simulink model "Damper_Bicycle_Output_Dec1"  (R2020a)
settings: Solver=ode4  StartTime=0.0  StopTime=2  FixedStep=0.0005  RelTol=1e-3  EnableMultiTasking=on
settings Model: Creator=Cason  LastModifiedBy=mjmck
settings SolverCC: AlgebraicLoopSolver=LineSearch

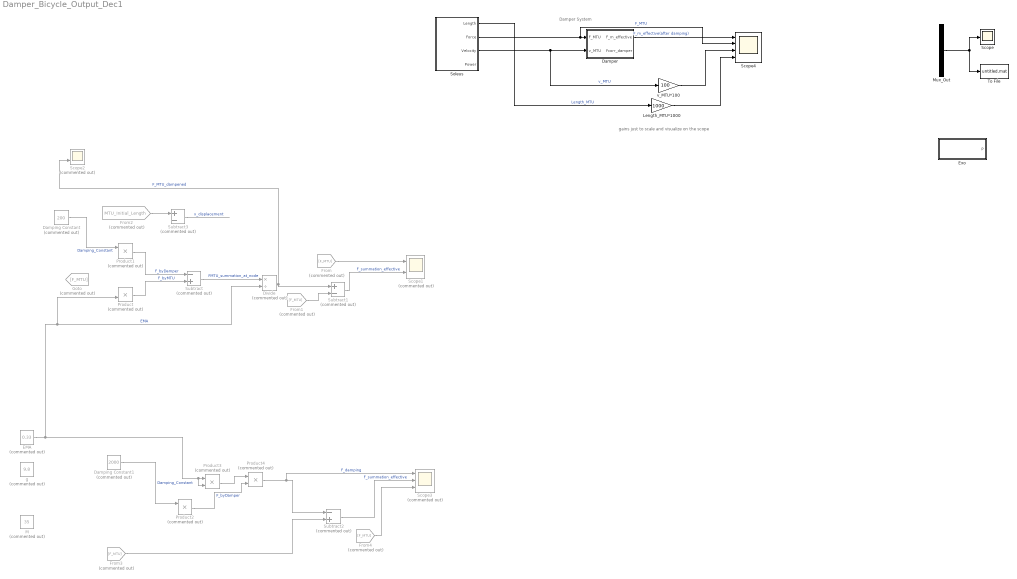
== system Damper_Bicycle_Output_Dec1 ==
  note: gains just to scale and visualize on the scope
  note: Damper System
  Damper : Subsystem
  Damping Constant : Constant  Commented=on  Value=200
  Damping Constant1 : Constant  Commented=on  Value=2000
  Divide : Product  Commented=on  Inputs=*/
  EMA : Constant  Commented=on  Value=0.33
  Exo : Subsystem
  From{,1,3..4} (4 alike) : From  Commented=on  GotoTag=F_MTU
  From2 : From  Commented=on  GotoTag=MTU_Initial_Length  TagVisibility=global
  Goto : Goto  Commented=on  GotoTag=F_MTU
  Length_MTU*1000 : Gain  Gain=1000
  M : Constant  Commented=on  Value=35
  Mux_Out : Mux
  Product{,1..4} (5 alike) : Product  Commented=on
  Scope : Scope
  Scope1 : Scope  Commented=on  NumInputPorts=2
  Scope2 : Scope  Commented=on  NumInputPorts=2
  Scope3 : Scope  Commented=on  NumInputPorts=3
  Scope4 : Scope  NumInputPorts=4
  Soleus : Subsystem
  Subtract : Sum  Commented=on  Inputs=-+
  Subtract1 : Sum  Commented=on  Inputs=+-
  Subtract2 : Sum  Commented=on  Inputs=-+
  Subtract3 : Sum  Commented=on  Inputs=+-
  To File : ToFile  MatrixName=out
  g : Constant  Commented=on  Value=9.8
  v_MTU*100 : Gain  Gain=100
  wires:
  Mux_Out/1 -> To File/1, Scope/1
  ? -> Scope2/1, Product/1, Goto/1  "F_MTU"
  EMA/1 -> Product3/2, Product3/1, Divide/2, Product/2  "EMA"
  Product/1 -> Subtract/2  "F_byMTU"
  ? -> Product2/2, Product1/2  "v_MTU"
  Product1/1 -> Subtract/1  "F_byDamper"
  Damping Constant/1 -> Product1/1  "Damping_Constant"
  Subtract/1 -> Divide/1  "FMTU_summation_at_node"
  Divide/1 -> Subtract1/1, Scope2/2  "F_MTU_dampened"
  From/1 -> Scope1/1
  From1/1 -> Subtract1/2
  Subtract1/1 -> Scope1/2  "F_summation_effective"
  ? -> Subtract3/2
  From2/1 -> Subtract3/1
  Subtract3/1 -> ?  "x_displacement"
  From3/1 -> Subtract2/2
  Damping Constant1/1 -> Product2/1  "Damping_Constant"
  Subtract2/1 -> Scope3/2  "F_summation_effective"
  From4/1 -> Scope3/3
  Product3/1 -> Product4/1
  Product2/1 -> Product4/2  "F_byDamper"
  Product4/1 -> Scope3/1, Subtract2/1  "F_damping"
  Soleus/3(Velocity) -> v_MTU*100/1, Damper/2(v_MTU)  "v_MTU"
  Soleus/2(Force) -> Scope4/2, Damper/1(F_MTU)  "F_MTU"
  Damper/1(F_m_effective) -> Scope4/1  "F_m_effective(after damping)"
  Soleus/1(Length) -> Length_MTU*1000/1  "Length_MTU"
  Length_MTU*1000/1 -> Scope4/4
  v_MTU*100/1 -> Scope4/3

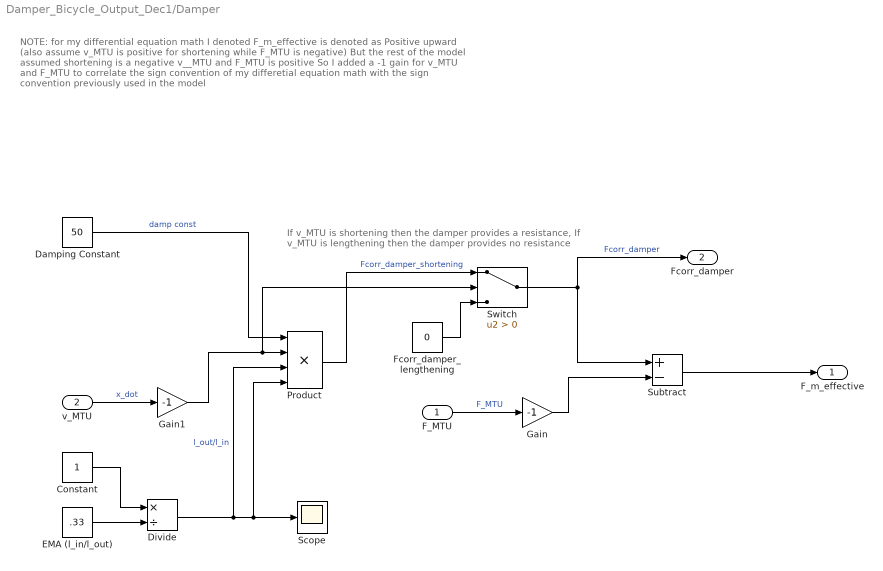
== system Damper_Bicycle_Output_Dec1/Damper ==
  note: NOTE:
      | for my differential equation math I denoted
      | 	F_m_effective is denoted as Positive upward (also assume v_MTU is positive for 			shortening while F_MTU is negative)
      |
      | But the rest of the model assumed shortening is a negative v__MTU and F_MTU is positive
      |
      | So I added a -1 gain for v_MTU and F_MTU to correlate the sign convention of my differetial equation math with the sign convention previously used in the model
  note: If v_MTU is shortening then the damper provides a resistance,
      | If v_MTU is lengthening then the damper provides no resistance
  F_MTU : Inport
  v_MTU : Inport  Port=2
  Constant : Constant
  Damping Constant : Constant  Value=50
  Divide : Product  Inputs=*/
  EMA (l_in/l_out) : Constant  Value=.33
  Fcorr_damper_lengthening : Constant  Value=0
  Gain : Gain  Gain=-1
  Gain1 : Gain  Gain=-1
  Product : Product  Inputs=4
  Scope : Scope
  Subtract : Sum  Inputs=+-
  Switch : Switch  Criteria=u2 > Threshold
  F_m_effective : Outport
  Fcorr_damper : Outport  Port=2
  wires:
  F_MTU/1 -> Gain/1  "F_MTU"
  Damping Constant/1 -> Product/1  "damp const"
  v_MTU/1 -> Gain1/1  "x_dot"
  EMA (l_in/l_out)/1 -> Divide/2
  Product/1 -> Switch/1  "Fcorr_damper_shortening"
  Constant/1 -> Divide/1
  Divide/1 -> Product/3, Product/4, Scope/1  "l_out/l_in"
  Switch/1 -> Fcorr_damper/1, Subtract/1  "Fcorr_damper"
  Fcorr_damper_lengthening/1 -> Switch/3
  Subtract/1 -> F_m_effective/1
  Gain/1 -> Subtract/2
  Gain1/1 -> Switch/2, Product/2

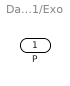
== system Damper_Bicycle_Output_Dec1/Exo ==
  P : Outport

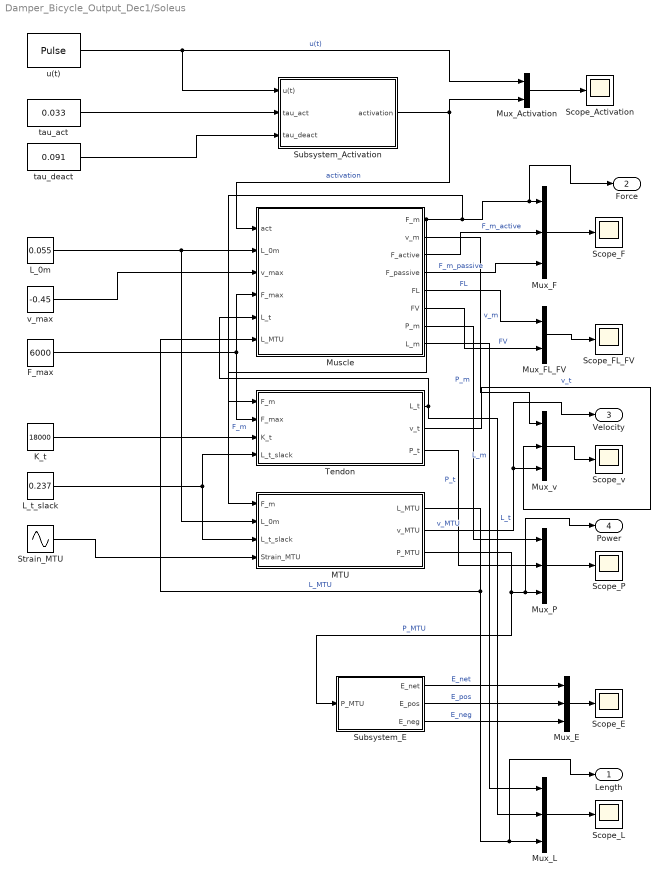
== system Damper_Bicycle_Output_Dec1/Soleus ==
  F_max : Constant  Value=6000
  K_t : Constant  Value=18000
  L_0m : Constant  Value=0.055
  L_t_slack : Constant  Value=0.237
  MTU : Subsystem
  Muscle : Subsystem
  Mux_Activation : Mux  Inputs=2
  Mux_E : Mux  Inputs=3
  Mux_F : Mux  Inputs=3
  Mux_FL_FV : Mux  Inputs=2
  Mux_L : Mux  Inputs=3
  Mux_P : Mux  Inputs=3
  Mux_v : Mux  Inputs=3
  Scope_Activation : Scope
  Scope_E : Scope
  Scope_F : Scope
  Scope_FL_FV : Scope
  Scope_L : Scope
  Scope_P : Scope
  Scope_v : Scope
  Strain_MTU : Sin  Amplitude=0.05  Bias=1  Frequency=5*pi  SampleTime=0
  Subsystem_Activation : Subsystem
  Subsystem_E : Subsystem
  Tendon : Subsystem
  tau_act : Constant  Value=0.033
  tau_deact : Constant  Value=0.091
  u(t) : DiscretePulseGenerator  PulseType=Time based  Period=0.4  PulseWidth=10
  v_max : Constant  Value=-0.45
  Length : Outport
  Force : Outport  Port=2
  Velocity : Outport  Port=3
  Power : Outport  Port=4
  wires:
  Mux_v/1 -> Scope_v/1
  u(t)/1 -> Mux_Activation/1, Subsystem_Activation/1(u(t))  "u(t)"
  Muscle/7(P_m) -> Mux_P/1  "P_m"
  tau_act/1 -> Subsystem_Activation/2(tau_act)
  K_t/1 -> Tendon/3(K_t)
  Mux_F/1 -> Scope_F/1
  MTU/3(P_MTU) -> Subsystem_E/1(P_MTU), Power/1, Mux_P/3  "P_MTU"
  Tendon/2(v_t) -> Mux_v/2  "v_t"
  L_t_slack/1 -> MTU/3(L_t_slack), Tendon/4(L_t_slack)
  MTU/1(L_MTU) -> Length/1, Mux_L/3, Muscle/6(L_MTU)  "L_MTU"
  Mux_P/1 -> Scope_P/1
  Tendon/1(L_t) -> Mux_L/2, Muscle/5(L_t)  "L_t"
  Mux_Activation/1 -> Scope_Activation/1
  MTU/2(v_MTU) -> Velocity/1, Mux_v/3  "v_MTU"
  Strain_MTU/1 -> MTU/4(Strain_MTU)
  Muscle/8(L_m) -> Mux_L/1  "L_m"
  Muscle/5(FL) -> Mux_FL_FV/1  "FL"
  v_max/1 -> Muscle/3(v_max)
  L_0m/1 -> MTU/2(L_0m), Muscle/2(L_0m)
  Muscle/6(FV) -> Mux_FL_FV/2  "FV"
  Tendon/3(P_t) -> Mux_P/2  "P_t"
  Muscle/4(F_passive) -> Mux_F/3  "F_m_passive"
  Muscle/2(v_m) -> Mux_v/1  "v_m"
  F_max/1 -> Tendon/2(F_max), Muscle/4(F_max)
  tau_deact/1 -> Subsystem_Activation/3(tau_deact)
  Mux_FL_FV/1 -> Scope_FL_FV/1
  Muscle/3(F_active) -> Mux_F/2  "F_m_active"
  Subsystem_Activation/1(activation) -> Mux_Activation/2, Muscle/1(act)  "activation"
  Mux_L/1 -> Scope_L/1
  Muscle/1(F_m) -> Tendon/1(F_m), MTU/1(F_m), Force/1, Mux_F/1  "F_m"
  Mux_E/1 -> Scope_E/1
  Subsystem_E/1(E_net) -> Mux_E/1  "E_net"
  Subsystem_E/2(E_pos) -> Mux_E/2  "E_pos"
  Subsystem_E/3(E_neg) -> Mux_E/3  "E_neg"

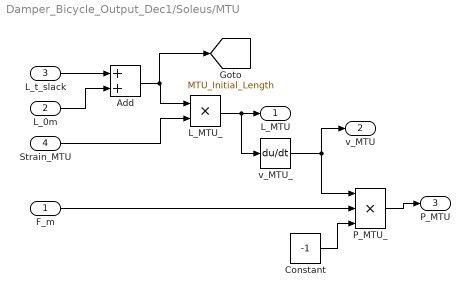
== system Damper_Bicycle_Output_Dec1/Soleus/MTU ==
  F_m : Inport
  L_0m : Inport  Port=2
  L_t_slack : Inport  Port=3
  Strain_MTU : Inport  Port=4
  Add : Sum
  Constant : Constant  Value=-1
  L_MTU_ : Product
  P_MTU_ : Product  Inputs=3
  v_MTU_ : Derivative
  L_MTU : Outport
  v_MTU : Outport  Port=2
  P_MTU : Outport  Port=3
  tag scope: MTU_Initial_Length=global
  wires:
  L_0m/1 -> Add/2
  v_MTU_/1 -> P_MTU_/1, v_MTU/1
  Strain_MTU/1 -> L_MTU_/2
  F_m/1 -> P_MTU_/2
  L_t_slack/1 -> Add/1
  L_MTU_/1 -> L_MTU/1, v_MTU_/1
  Add/1 -> [MTU_Initial_Length], L_MTU_/1
  P_MTU_/1 -> P_MTU/1
  Constant/1 -> P_MTU_/3

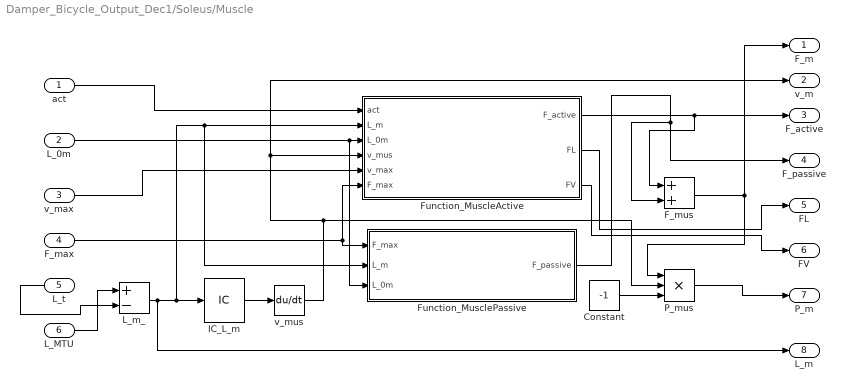
== system Damper_Bicycle_Output_Dec1/Soleus/Muscle ==
  act : Inport
  L_0m : Inport  Port=2
  v_max : Inport  Port=3
  F_max : Inport  Port=4
  L_t : Inport  Port=5
  L_MTU : Inport  Port=6
  Constant : Constant  Value=-1
  F_mus : Sum
  Function_MuscleActive : MATLAB Function  TreatAsAtomicUnit=on
  Function_MusclePassive : MATLAB Function  TreatAsAtomicUnit=on
  IC_L_m : InitialCondition  Value=0.055
  L_m_ : Sum  Inputs=+-
  P_mus : Product  Inputs=3
  v_mus : Derivative
  F_m : Outport
  v_m : Outport  Port=2
  F_active : Outport  Port=3
  F_passive : Outport  Port=4
  FL : Outport  Port=5
  FV : Outport  Port=6
  P_m : Outport  Port=7
  L_m : Outport  Port=8
  wires:
  L_t/1 -> L_m_/2
  IC_L_m/1 -> v_mus/1
  Function_MusclePassive/1(F_passive) -> F_passive/1, F_mus/2
  L_m_/1 -> L_m/1, IC_L_m/1, Function_MusclePassive/2(L_m), Function_MuscleActive/2(L_m)
  L_0m/1 -> Function_MusclePassive/3(L_0m), Function_MuscleActive/3(L_0m)
  v_mus/1 -> v_m/1, Function_MuscleActive/4(v_mus), P_mus/2
  Function_MuscleActive/2(FL) -> FL/1
  Function_MuscleActive/1(F_active) -> F_mus/1, F_active/1
  act/1 -> Function_MuscleActive/1(act)
  v_max/1 -> Function_MuscleActive/5(v_max)
  F_mus/1 -> F_m/1, P_mus/1
  F_max/1 -> Function_MuscleActive/6(F_max), Function_MusclePassive/1(F_max)
  P_mus/1 -> P_m/1
  Function_MuscleActive/3(FV) -> FV/1
  Constant/1 -> P_mus/3
  L_MTU/1 -> L_m_/1

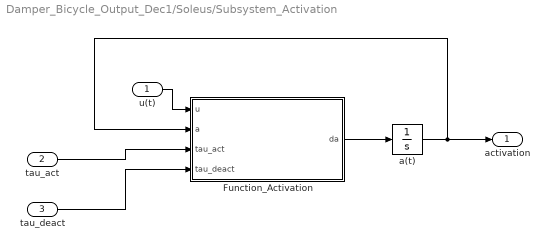
== system Damper_Bicycle_Output_Dec1/Soleus/Subsystem_Activation ==
  u(t) : Inport
  tau_act : Inport  Port=2
  tau_deact : Inport  Port=3
  Function_Activation : MATLAB Function  TreatAsAtomicUnit=on
  a(t) : Integrator
  activation : Outport
  wires:
  Function_Activation/1(da) -> a(t)/1
  tau_deact/1 -> Function_Activation/4(tau_deact)
  tau_act/1 -> Function_Activation/3(tau_act)
  a(t)/1 -> Function_Activation/2(a), activation/1
  u(t)/1 -> Function_Activation/1(u)

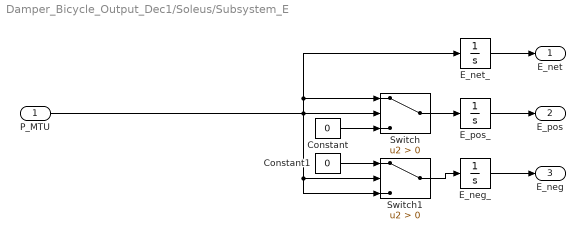
== system Damper_Bicycle_Output_Dec1/Soleus/Subsystem_E ==
  P_MTU : Inport
  Constant : Constant  Value=0
  Constant1 : Constant  Value=0
  E_neg_ : Integrator
  E_net_ : Integrator
  E_pos_ : Integrator
  Switch : Switch  Criteria=u2 > Threshold
  Switch1 : Switch  Criteria=u2 > Threshold
  E_net : Outport
  E_pos : Outport  Port=2
  E_neg : Outport  Port=3
  wires:
  Constant/1 -> Switch/3
  E_pos_/1 -> E_pos/1
  Constant1/1 -> Switch1/1
  P_MTU/1 -> Switch1/3, Switch1/2, Switch/2, E_net_/1, Switch/1
  Switch/1 -> E_pos_/1
  Switch1/1 -> E_neg_/1
  E_neg_/1 -> E_neg/1
  E_net_/1 -> E_net/1

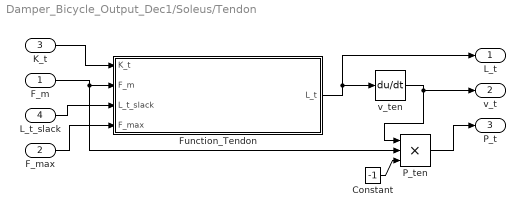
== system Damper_Bicycle_Output_Dec1/Soleus/Tendon ==
  F_m : Inport
  F_max : Inport  Port=2
  K_t : Inport  Port=3
  L_t_slack : Inport  Port=4
  Constant : Constant  Value=-1
  Function_Tendon : MATLAB Function  TreatAsAtomicUnit=on
  P_ten : Product  Inputs=3
  v_ten : Derivative
  L_t : Outport
  v_t : Outport  Port=2
  P_t : Outport  Port=3
  wires:
  Constant/1 -> P_ten/3
  F_m/1 -> P_ten/2, Function_Tendon/2(F_m)
  L_t_slack/1 -> Function_Tendon/3(L_t_slack)
  F_max/1 -> Function_Tendon/4(F_max)
  K_t/1 -> Function_Tendon/1(K_t)
  v_ten/1 -> P_ten/1, v_t/1
  P_ten/1 -> P_t/1
  Function_Tendon/1(L_t) -> L_t/1, v_ten/1

== matlab function Damper_Bicycle_Output_Dec1/Soleus/Muscle/Function_MuscleActive ==
  data: act input; F_active output; L_m input; L_0m input; v_mus input; v_max input; F_max input; FL output; FV output
function [F_active, FL, FV]= active_muscle_dynamics(act, L_m, L_0m, v_mus, v_max, F_max)
a = 3.1108; b = 0.8698; s = 0.3914;

if L_m < 0
    L_m = 0;
end

FL = exp(-abs(((L_m / L_0m)^b - 1) / s)^a);

if v_mus < v_max
    FV = 0;
elseif v_mus >= v_max && v_mus < 0  % Shortening
    FV = (1 - v_mus/v_max) / (1 + v_mus/(0.17*v_max));
else                                % Lengthening
    FV = 1.8 - 0.8*((1 + v_mus/v_max) / (1 - 7.56*(v_mus/(0.17*v_max))));
end

F_active = act * FL * FV * F_max;

== matlab function Damper_Bicycle_Output_Dec1/Soleus/Subsystem_Activation/Function_Activation ==
  data: u input; da output; a input; tau_act input; tau_deact input
function da = activation(u, a, tau_act, tau_deact)
beta = tau_act / tau_deact;
da = u / tau_act - (beta + (1 - beta)*u) / tau_act * a;

== matlab function Damper_Bicycle_Output_Dec1/Soleus/Muscle/Function_MusclePassive ==
  data: F_max input; F_passive output; L_m input; L_0m input
function F_passive = passive_muscle_dynamics(F_max, L_m, L_0m)
A = 2.39E-2; b = 5.31;

F_passive = F_max*A*exp(b*(L_m/L_0m - 1));

== matlab function Damper_Bicycle_Output_Dec1/Soleus/Tendon/Function_Tendon ==
  data: K_t input; L_t output; F_m input; L_t_slack input; F_max input
function L_t = tendon_dynamics(K_t, F_m, L_t_slack, F_max)
D_L_t = (F_m + (F_max*log(-9*exp(-(20*F_m)/F_max)+ 10)) / 20) / K_t;
L_t = D_L_t + L_t_slack;
